simulink model "autonomous_vehicle"  (R2026a)
settings: Solver=VariableStepAuto
values from neighbouring files (symbols this model uses):
  b = 2e-5    (= 2e-05)    [init_parameters.m]
  J = 2e-5    (= 2e-05)    [init_parameters.m]
  Ke = 0.02    [init_parameters.m]
  Kt = 0.02    [init_parameters.m]
  L = 2e-3    (= 0.002)    [init_parameters.m]
  R = 4    [init_parameters.m]
settings Model: Creator=aliad  LastModifiedBy=aliad

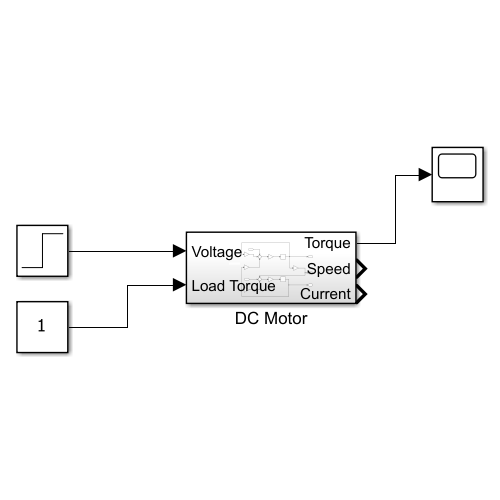
[thumbnail: Simulink's stored preview of the top-level diagram]
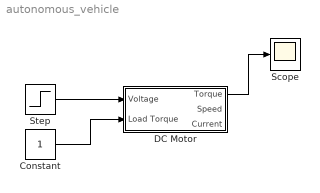
== system autonomous_vehicle ==
  Constant : Constant
  DC Motor : Subsystem
  Scope : Scope
  Step : Step  SampleTime=0
  wires:
  DC Motor/1(" Torque") -> Scope/1
  Step/1 -> DC Motor/1(Voltage)
  Constant/1 -> DC Motor/2(Load Torque)

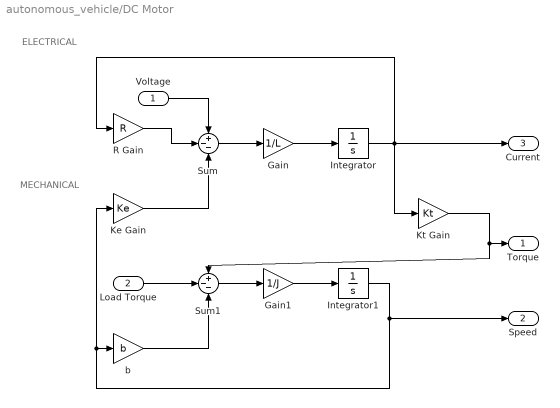
== system autonomous_vehicle/DC Motor ==
  note: ELECTRICAL
  note: MECHANICAL
  Voltage : Inport
  Load Torque : Inport  Port=2
  Gain : Gain  Gain=1/L
  Gain1 : Gain  Gain=1/J
  Integrator : Integrator
  Integrator1 : Integrator
  Ke Gain : Gain  Gain=Ke
  Kt Gain : Gain  Gain=Kt
  R Gain : Gain  Gain=R
  Sum : Sum  Inputs=+--
  Sum1 : Sum  Inputs=+--
  b : Gain  Gain=b
  " Torque" : Outport
  Speed : Outport  Port=2
  Current : Outport  Port=3
  wires:
  R Gain/1 -> Sum/2
  Integrator1/1 -> Speed/1, Ke Gain/1, b/1
  Kt Gain/1 -> " Torque"/1, Sum1/1
  Gain1/1 -> Integrator1/1
  Integrator/1 -> Kt Gain/1, Current/1, R Gain/1
  Load Torque/1 -> Sum1/2
  Gain/1 -> Integrator/1
  Ke Gain/1 -> Sum/3
  Sum/1 -> Gain/1
  Sum1/1 -> Gain1/1
  Voltage/1 -> Sum/1
  b/1 -> Sum1/3
